simulink model "demo1"  (Simulink 7.1)
settings: Solver=ode3  StartTime=0.0  StopTime=10.0  RelTol=1e-3
libraries: roblocks x2, simulink x1
settings Model: Creator=pic  LastModifiedBy=pic  ExtModeTrigMode=oneshot  ExtModeArmWhenConnect=off
settings DataIOCC: LimitDataPoints=off
settings OptimizationCC: BlockReduction=off  BooleanDataType=off
settings DebuggingCC: SaveWithParameterizedLinksMsg=none  SignalResolutionControl=TryResolveAllWithWarning  SolverPrmCheckMsg=none  MultiTaskDSMMsg=warning  MultiTaskCondExecSysMsg=none  StrictBusMsg=None
settings HardwareCC: TargetUnknown=on
settings RTWCC: IncludeERTFirstTime=on
settings STFCustomTargetCC: ModelReferenceCompliant=off  SystemTargetFile=grt.tlc

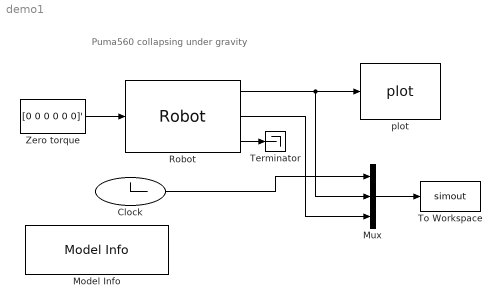
== system demo1 ==
  note: Puma560 collapsing under gravity
  Clock : Clock
  Model Info : simulink/Model-Wide Utilities/Model Info  SystemSampleTime=-1  InitialBlockCM=none  BlockCM=none  Frame=on  DisplayStringWithTags=|  HorizontalTextAlignment=Left  LeftAlignmentValue=0.02  SourceBlockDiagram=demo1  TagMaxNumber=20
      | Simple dynamics demo
      | %<Creator>
      | %<LastModificationDate>
  Mux : Mux  Inputs=3
  Robot : roblocks/Robot  SystemSampleTime=-1  robot=p560  q0=[0 0 0 0 0 0]
  Terminator : Terminator
  To Workspace : ToWorkspace  VariableName=simout  SampleTime=-1  SaveFormat=Array
  Zero torque : Constant  Value=[0 0 0 0 0 0]'
  plot : roblocks/plot  SystemSampleTime=-1  robot=p560
  wires:
  Zero torque/1 -> Robot/1
  Mux/1 -> To Workspace/1
  Robot/1 -> plot/1, Mux/2
  Clock/1 -> Mux/1
  Robot/2 -> Mux/3
  Robot/3 -> Terminator/1
